simulink model "pmsm_mpc_ekf"  (R2025b)
settings: Solver=ode23tb  StartTime=0.0  StopTime=simlength  FixedStep=tsample  MaxStep=ts
undefined symbols (not defined in the file): A1_tilde, A2_tilde, A3_tilde, A4_tilde, Adrso, b, b_brake, Bd, C, Crso, ibez, Jm, ki_w, kp_w, Lalpha, Lbeta, Ldrso, omega_bez, omega_m_bez, omega_m_sim, psi_m, Qkalman, Rkalman, Rs, simlength, tau_bez, tcontrol, ts, Vdc
libraries: fl_lib x19, nesl_utility x19, pmsm_alphabeta_lib x1, psm x1
(part 1 of 2)
settings Model: SimulationMode=accelerator  Creator=dbagn  LastModifiedBy=dbagn
settings SolverCC: NumberNewtonIterations=3.0  ZeroCrossControl=DisableAll  AlgebraicLoopSolver=TrustRegion  SolverResetMethod=Robust
settings DataIOCC: ReturnWorkspaceOutputs=off
settings DebuggingCC: UnconnectedInputMsg=warning  UnconnectedOutputMsg=warning  UnconnectedLineMsg=warning
settings ModelReferenceCC: EnableRefExpFcnMdlSchedulingChecks=on
settings RTWCC: GPUComputeCapability=3.5  DLArmComputeVersion=19.05

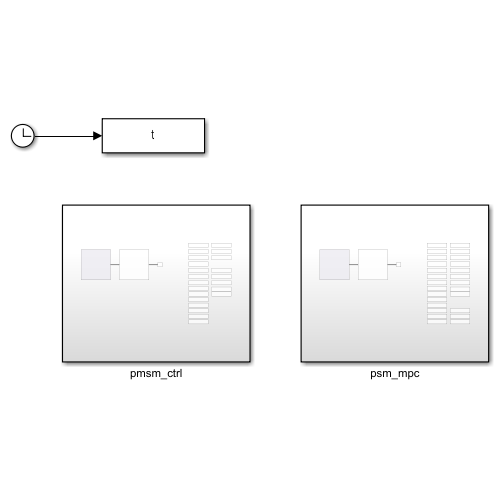
[thumbnail: Simulink's stored preview of the top-level diagram]
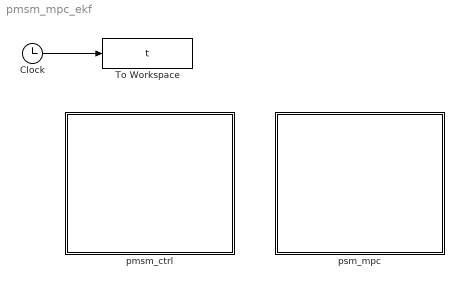
== system pmsm_mpc_ekf ==
  Clock : Clock
  To Workspace : ToWorkspace  VariableName=t  SampleTime=ts
      settings: MaxDataPoints=Nc
  pmsm_ctrl : Subsystem
  psm_mpc : Subsystem
  wires:
  Clock/1 -> To Workspace/1

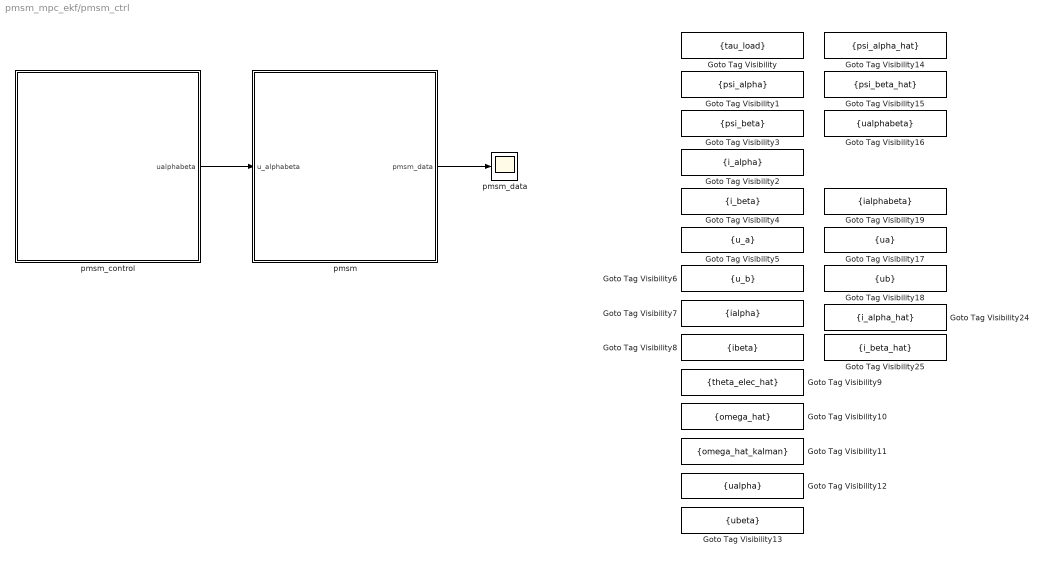
== system pmsm_mpc_ekf/pmsm_ctrl ==
  Goto Tag Visibility : GotoTagVisibility  GotoTag=tau_load
  Goto Tag Visibility1 : GotoTagVisibility  GotoTag=psi_alpha
  Goto Tag Visibility10 : GotoTagVisibility  GotoTag=omega_hat
  Goto Tag Visibility11 : GotoTagVisibility  GotoTag=omega_hat_kalman
  Goto Tag Visibility12 : GotoTagVisibility  GotoTag=ualpha
  Goto Tag Visibility13 : GotoTagVisibility  GotoTag=ubeta
  Goto Tag Visibility14 : GotoTagVisibility  GotoTag=psi_alpha_hat
  Goto Tag Visibility15 : GotoTagVisibility  GotoTag=psi_beta_hat
  Goto Tag Visibility16 : GotoTagVisibility  GotoTag=ualphabeta
  Goto Tag Visibility17 : GotoTagVisibility  GotoTag=ua
  Goto Tag Visibility18 : GotoTagVisibility  GotoTag=ub
  Goto Tag Visibility19 : GotoTagVisibility  GotoTag=ialphabeta
  Goto Tag Visibility2 : GotoTagVisibility  GotoTag=i_alpha
  Goto Tag Visibility24 : GotoTagVisibility  GotoTag=i_alpha_hat
  Goto Tag Visibility25 : GotoTagVisibility  GotoTag=i_beta_hat
  Goto Tag Visibility3 : GotoTagVisibility  GotoTag=psi_beta
  Goto Tag Visibility4 : GotoTagVisibility  GotoTag=i_beta
  Goto Tag Visibility5 : GotoTagVisibility  GotoTag=u_a
  Goto Tag Visibility6 : GotoTagVisibility  GotoTag=u_b
  Goto Tag Visibility7 : GotoTagVisibility  GotoTag=ialpha
  Goto Tag Visibility8 : GotoTagVisibility  GotoTag=ibeta
  Goto Tag Visibility9 : GotoTagVisibility  GotoTag=theta_elec_hat
  pmsm : Subsystem
  pmsm_control : Subsystem
  pmsm_data : Scope
      settings: ActiveDisplayYMinimum=-7553.3407677630657  ActiveDisplayYMaximum=8430.65022613591
  wires:
  pmsm_control/1(ualphabeta) -> pmsm/1(u_alphabeta)
  pmsm/1(pmsm_data) -> pmsm_data/1

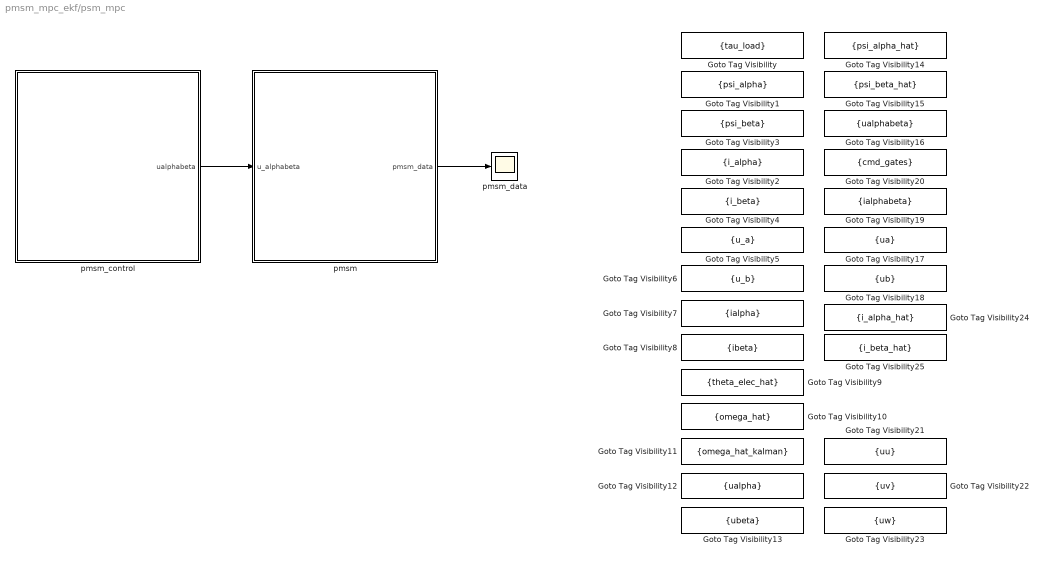
== system pmsm_mpc_ekf/psm_mpc ==
  Goto Tag Visibility : GotoTagVisibility  GotoTag=tau_load
  Goto Tag Visibility1 : GotoTagVisibility  GotoTag=psi_alpha
  Goto Tag Visibility10 : GotoTagVisibility  GotoTag=omega_hat
  Goto Tag Visibility11 : GotoTagVisibility  GotoTag=omega_hat_kalman
  Goto Tag Visibility12 : GotoTagVisibility  GotoTag=ualpha
  Goto Tag Visibility13 : GotoTagVisibility  GotoTag=ubeta
  Goto Tag Visibility14 : GotoTagVisibility  GotoTag=psi_alpha_hat
  Goto Tag Visibility15 : GotoTagVisibility  GotoTag=psi_beta_hat
  Goto Tag Visibility16 : GotoTagVisibility  GotoTag=ualphabeta
  Goto Tag Visibility17 : GotoTagVisibility  GotoTag=ua
  Goto Tag Visibility18 : GotoTagVisibility  GotoTag=ub
  Goto Tag Visibility19 : GotoTagVisibility  GotoTag=ialphabeta
  Goto Tag Visibility2 : GotoTagVisibility  GotoTag=i_alpha
  Goto Tag Visibility20 : GotoTagVisibility  GotoTag=cmd_gates
  Goto Tag Visibility21 : GotoTagVisibility  GotoTag=uu
  Goto Tag Visibility22 : GotoTagVisibility  GotoTag=uv
  Goto Tag Visibility23 : GotoTagVisibility  GotoTag=uw
  Goto Tag Visibility24 : GotoTagVisibility  GotoTag=i_alpha_hat
  Goto Tag Visibility25 : GotoTagVisibility  GotoTag=i_beta_hat
  Goto Tag Visibility3 : GotoTagVisibility  GotoTag=psi_beta
  Goto Tag Visibility4 : GotoTagVisibility  GotoTag=i_beta
  Goto Tag Visibility5 : GotoTagVisibility  GotoTag=u_a
  Goto Tag Visibility6 : GotoTagVisibility  GotoTag=u_b
  Goto Tag Visibility7 : GotoTagVisibility  GotoTag=ialpha
  Goto Tag Visibility8 : GotoTagVisibility  GotoTag=ibeta
  Goto Tag Visibility9 : GotoTagVisibility  GotoTag=theta_elec_hat
  pmsm : Subsystem
  pmsm_control : Subsystem
  pmsm_data : Scope
      settings: ActiveDisplayYMinimum=-7553.3407677630657  ActiveDisplayYMaximum=8430.65022613591
  wires:
  pmsm/1(pmsm_data) -> pmsm_data/1
  pmsm_control/1(ualphabeta) -> pmsm/1(u_alphabeta)

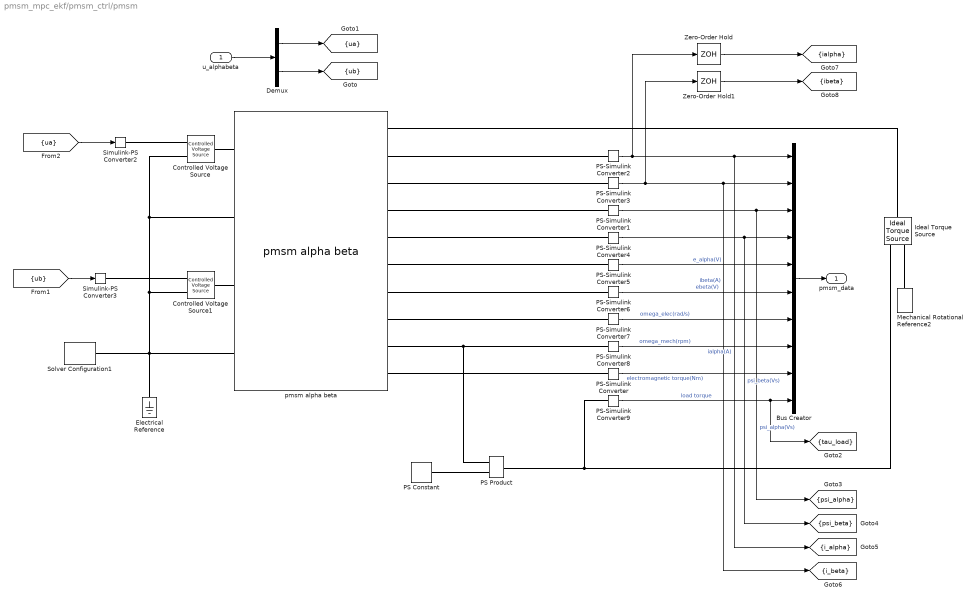
== system pmsm_mpc_ekf/pmsm_ctrl/pmsm ==
  u_alphabeta : Inport
  Bus Creator : BusCreator  Inputs=10
  Controlled Voltage Source : fl_lib/Electrical/Electrical Sources/Controlled Voltage Source
  Controlled Voltage Source1 : fl_lib/Electrical/Electrical Sources/Controlled Voltage Source
  Demux : Demux  Outputs=2
  Electrical Reference : fl_lib/Electrical/Electrical Elements/Electrical Reference
  Ideal Torque Source : fl_lib/Mechanical/Mechanical Sources/Ideal Torque Source
  Mechanical Rotational Reference2 : fl_lib/Mechanical/Rotational Elements/Mechanical Rotational Reference
  PS Constant : fl_lib/Physical Signals/Sources/PS Constant  constant=-b_brake N*m/(rad/s)
  PS Product : fl_lib/Physical Signals/Functions/PS Product
  PS-Simulink Converter : nesl_utility/PS-Simulink Converter  PhysicalDomain=network_engine_domain  SubClassName=ps_output  LeftPortType=input  RightPortType=output  PseudoPeriodic=off  Frequencies=[]  VectorFormat=1-D array  Unit=N*m  AffineConversion=on
  PS-Simulink Converter1 : nesl_utility/PS-Simulink Converter  PhysicalDomain=network_engine_domain  SubClassName=ps_output  LeftPortType=input  RightPortType=output  PseudoPeriodic=off  Frequencies=[]  VectorFormat=1-D array  Unit=V*s  AffineConversion=on
  PS-Simulink Converter2 : nesl_utility/PS-Simulink Converter  PhysicalDomain=network_engine_domain  SubClassName=ps_output  LeftPortType=input  RightPortType=output  PseudoPeriodic=off  Frequencies=[]  VectorFormat=1-D array  Unit=A  AffineConversion=on
  PS-Simulink Converter3 : nesl_utility/PS-Simulink Converter  PhysicalDomain=network_engine_domain  SubClassName=ps_output  LeftPortType=input  RightPortType=output  PseudoPeriodic=off  Frequencies=[]  VectorFormat=1-D array  Unit=A  AffineConversion=on
  PS-Simulink Converter4 : nesl_utility/PS-Simulink Converter  PhysicalDomain=network_engine_domain  SubClassName=ps_output  LeftPortType=input  RightPortType=output  PseudoPeriodic=off  Frequencies=[]  VectorFormat=1-D array  Unit=V*s  AffineConversion=on
  PS-Simulink Converter5 : nesl_utility/PS-Simulink Converter  PhysicalDomain=network_engine_domain  SubClassName=ps_output  LeftPortType=input  RightPortType=output  PseudoPeriodic=off  Frequencies=[]  VectorFormat=1-D array  Unit=V  AffineConversion=on
  PS-Simulink Converter6 : nesl_utility/PS-Simulink Converter  PhysicalDomain=network_engine_domain  SubClassName=ps_output  LeftPortType=input  RightPortType=output  PseudoPeriodic=off  Frequencies=[]  VectorFormat=1-D array  Unit=V  AffineConversion=on
  PS-Simulink Converter7 : nesl_utility/PS-Simulink Converter  PhysicalDomain=network_engine_domain  SubClassName=ps_output  LeftPortType=input  RightPortType=output  PseudoPeriodic=off  Frequencies=[]  VectorFormat=1-D array  Unit=rad/s  AffineConversion=on
  PS-Simulink Converter8 : nesl_utility/PS-Simulink Converter  PhysicalDomain=network_engine_domain  SubClassName=ps_output  LeftPortType=input  RightPortType=output  PseudoPeriodic=off  Frequencies=[]  VectorFormat=1-D array  Unit=rpm  AffineConversion=on
  PS-Simulink Converter9 : nesl_utility/PS-Simulink Converter  PhysicalDomain=network_engine_domain  SubClassName=ps_output  LeftPortType=input  RightPortType=output  PseudoPeriodic=off  Frequencies=[]  VectorFormat=1-D array  Unit=N*m  AffineConversion=on
  Simulink-PS Converter2 : nesl_utility/Simulink-PS Converter  PhysicalDomain=network_engine_domain  SubClassName=ps_input  LeftPortType=input  RightPortType=output  PseudoPeriodic=off  Frequencies=[]  NoiseDistribution=none  NoiseParameters=[]  Unit=1  AffineConversion=off  FilteringAndDerivatives=provide  SimscapeFilterOrder=1  InputFilterTimeConstant=0.001  UdotUserProvided=0
  Simulink-PS Converter3 : nesl_utility/Simulink-PS Converter  PhysicalDomain=network_engine_domain  SubClassName=ps_input  LeftPortType=input  RightPortType=output  PseudoPeriodic=off  Frequencies=[]  NoiseDistribution=none  NoiseParameters=[]  Unit=1  AffineConversion=off  FilteringAndDerivatives=provide  SimscapeFilterOrder=1  InputFilterTimeConstant=0.001  UdotUserProvided=0
  Solver Configuration1 : nesl_utility/Solver Configuration  PhysicalDomain=network_engine_domain  SubClassName=solver  LeftPortType=input  RightPortType=generic  Tones=[]  Harmonics=[]  SimulateNoise=off  Profile=off  UseLocalSampling=off  EnableSwitchedLinearOptims=on  FrequencyDomain=off  UseCCode=off  RelTol=0.001  AbsTol=1e-06  MinStep=1e-09  ToWorkspace=off  RevertToSquareIcSolve=off  NumHomotopyIterations=100  PhasorMode=off  PhasorModeNumHarmonics=1  ConsistencySolver=NEWTON_FTOL  IndexReductionMethod=DerivativeReplacement  DoDC=on  ResidualTolerance=1e-09  ConsistencyTolSource=GLOBAL  ConsistencyAbsTol=0.001  ConsistencyRelTol=0.001  ConsistencyTolFactor=0.001  UseLocalSolver=on  LocalSolverChoice=NE_TRAPEZOIDAL_ADVANCER  ResolveIndetEquations=on  FunctionEvalNumThread=1  LocalSolverSampleTime=ts  DoFixedCost=on  MaxNonlinIter=3  MaxModeIter=2  ComputeImpulses=off  ImpulseIterations=2  LinearAlgebra=auto  LinearAlgebraNumThread=0  EquationFormulation=NE_TIME_EF  DelaysMemoryBudget=1024*4  AutomaticFiltering=on  FilteringTimeConstant=ts  PartitionStorageMethod=AS_NEEDED  PartitionMemoryBudget=1024  PartitionMethod=ROBUST  MultibodyUseLocalSolver=off  MultibodyLocalSolverChoice=ODE1  MultibodyLocalSolverSampleTime=0.001
  Zero-Order Hold : ZeroOrderHold  SampleTime=tcontrol
  Zero-Order Hold1 : ZeroOrderHold  SampleTime=tcontrol
  pmsm alpha beta : pmsm_alphabeta_lib/pmsm alpha beta  number_poles=number_poles  psi_m=psi_m V*s  Ls=Ls H  Lb=Lb H  Rs=Rs Ohm  J=Jm kg*m^2  b=b N*m/(rad/s)  omega_specify=off  omega_priority=None  omega=0 rad/s  omega_nominal_specify=off  omega_nominal_unit=rad/s  omega_nominal_value=1  omega_m_specify=off  omega_m_priority=None  omega_m=0 rad/s  omega_m_nominal_specify=off  omega_m_nominal_unit=rad/s  omega_m_nominal_value=1  ialpha_specify=on  ialpha_priority=High  ialpha=0 A  ialpha_nominal_specify=off  ialpha_nominal_unit=A  ialpha_nominal_value=1  ualpha_specify=off  ualpha_priority=None  ualpha=0 V  ualpha_nominal_specify=off  ualpha_nominal_unit=V  ualpha_nominal_value=1  psi_beta_specify=off  psi_beta_priority=High  psi_beta=0.0 V*s  psi_beta_nominal_specify=off  psi_beta_nominal_unit=V*s  psi_beta_nominal_value=1  ibeta_specify=on  ibeta_priority=High  ibeta=0 A  ibeta_nominal_specify=off  ibeta_nominal_unit=A  ibeta_nominal_value=1  ubeta_specify=off  ubeta_priority=None  ubeta=0 V  ubeta_nominal_specify=off  ubeta_nominal_unit=V  ubeta_nominal_value=1  tau_load_specify=off  tau_load_priority=None  tau_load=0 N*m  tau_load_nominal_specify=off  tau_load_nominal_unit=N*m  tau_load_nominal_value=1
      settings: InternalSimscapePortConfiguration="{\"Bottom\":[],\"Left\":[{\"id\":\"u_alpha_p\",\"label\":\"_u_alpha+_\",\"type\":\"foundation.electrical.electrical\"},{\"id\":\"u_alpha_n\",\"label\":\"_u_alpha-_\",\"type\":\"foundation.electrical.electrical\"},{\"id\":\"u_beta_p\",\"label\":\"_u_beta+_\",\"type\":\"foundation.electrical.electrical\"},{\"id\":\"u_beta_n\",\"label\":\"_u_beta-_\",\"type\":\"foundation.electrical.electrical\"}],\"Right\":[{\"id\":\"s\",\"label\":\"_s_\",\"type\":\"foundation.mechanical.rotational.rotational\"},{\"id\":\"i_alpha_out\",\"label\":\"_i_alpha_\",\"type\":\"output\"},{\"id\":\"i_beta_out\",\"label\":\"_i_beta_\",\"type\":\"output\"},{\"id\":\"psi_alpha_out\",\"label\":\"_psi_alpha_\",\"type\":\"output\"},{\"id\":\"psi_beta_out\",\"label\":\"_psi_beta_\",\"type\":\"output\"},{\"id\":\"e_alpha_out\",\"label\":\"_e_alpha_\",\"type\":\"output\"},{\"id\":\"e_beta_out\",\"label\":\"_e_beta_\",\"type\":\"output\"},{\"id\":\"omega_elec_out\",\"label\":\"_omega_elec_\",\"type\":\"output\"},{\"id\":\"omega_mech_out\",\"label\":\"_omega_mech_\",\"type\":\"output\"},{\"id\":\"torque_e_out\",\"label\":\"_torque_e_\",\"type\":\"output\"}],\"Top\":[]}"
  pmsm_data : Outport
  tag scope: i_alpha=scoped, i_beta=scoped, ialpha=scoped, ibeta=scoped, psi_alpha=scoped, psi_beta=scoped, tau_load=scoped, ua=scoped, ub=scoped
  wires:
  [ua] -> Simulink-PS Converter2/1
  [ub] -> Simulink-PS Converter3/1
  u_alphabeta/1 -> Demux/1
  Demux/1 -> [ua]
  Demux/2 -> [ub]
  Zero-Order Hold/1 -> [ialpha]
  Zero-Order Hold1/1 -> [ibeta]
  PS-Simulink Converter2/1 -> [i_alpha], Bus Creator/1, Zero-Order Hold/1  "ialpha(A)"
  PS-Simulink Converter3/1 -> [i_beta], Bus Creator/2, Zero-Order Hold1/1  "ibeta(A)"
  PS-Simulink Converter1/1 -> [psi_alpha], Bus Creator/3  "psi_alpha(Vs)"
  PS-Simulink Converter4/1 -> Bus Creator/4, [psi_beta]  "psi_beta(Vs)"
  PS-Simulink Converter5/1 -> Bus Creator/5  "e_alpha(V)"
  PS-Simulink Converter6/1 -> Bus Creator/6  "ebeta(V)"
  PS-Simulink Converter7/1 -> Bus Creator/7  "omega_elec(rad/s)"
  PS-Simulink Converter8/1 -> Bus Creator/8  "omega_mech(rpm)"
  PS-Simulink Converter/1 -> Bus Creator/9  "electromagnetic torque(Nm)"
  PS-Simulink Converter9/1 -> Bus Creator/10, [tau_load]  "load torque"
  Bus Creator/1 -> pmsm_data/1
  connections:
  Controlled Voltage Source/RConn1 -- Simulink-PS Converter2/RConn1
  pmsm alpha beta/LConn1 -- Controlled Voltage Source/LConn1
  Simulink-PS Converter3/RConn1 -- Controlled Voltage Source1/RConn1
  pmsm alpha beta/LConn3 -- Controlled Voltage Source1/LConn1
  Controlled Voltage Source/RConn2 -- pmsm alpha beta/LConn2 -- Controlled Voltage Source1/RConn2 -- pmsm alpha beta/LConn4 -- Solver Configuration1/RConn1 -- Electrical Reference/LConn1
  pmsm alpha beta/RConn2 -- PS-Simulink Converter2/LConn1
  pmsm alpha beta/RConn3 -- PS-Simulink Converter3/LConn1
  PS-Simulink Converter4/LConn1 -- pmsm alpha beta/RConn5
  PS-Simulink Converter1/LConn1 -- pmsm alpha beta/RConn4
  PS-Simulink Converter5/LConn1 -- pmsm alpha beta/RConn6
  pmsm alpha beta/RConn7 -- PS-Simulink Converter6/LConn1
  Mechanical Rotational Reference2/LConn1 -- Ideal Torque Source/RConn2
  pmsm alpha beta/RConn1 -- Ideal Torque Source/LConn1
  pmsm alpha beta/RConn9 -- PS-Simulink Converter8/LConn1 -- PS Product/LConn1
  pmsm alpha beta/RConn10 -- PS-Simulink Converter/LConn1
  PS Constant/RConn1 -- PS Product/LConn2
  PS Product/RConn1 -- Ideal Torque Source/RConn1 -- PS-Simulink Converter9/LConn1
  pmsm alpha beta/RConn8 -- PS-Simulink Converter7/LConn1

== system pmsm_mpc_ekf/pmsm_ctrl/pmsm_control ==
  Mux : Mux  Inputs=2
  Speed control : Subsystem
  double_integrator_observer : Subsystem
  mpc_ekf : Subsystem
  normalization : Gain  Gain=1/omega_bez
  normalization1 : Gain  Gain=1/tau_bez
  omega_hat_kalman/omega_hat : Scope  NumInputPorts=2
      settings: SampleTime=tcontrol  ActiveDisplayYMinimum=-304.159  ActiveDisplayYMaximum=313.10699
  omega_ref/omega/torque load_pu : Scope  NumInputPorts=2
      settings: SampleTime=tcontrol  ActiveDisplayYMinimum=-1.08049  ActiveDisplayYMaximum=1.23758  DataLoggingVariableName=ScopeData3
  speed_reference_generator : Subsystem
  torque_ref_pu : Scope
      settings: SampleTime=tcontrol  ActiveDisplayYMinimum=-1.08049  ActiveDisplayYMaximum=1.23758
  ualphabeta : Outport  VectorParamsAs1DForOutWhenUnconnected=off
  tag scope: omega_hat=scoped
  wires:
  mpc_ekf/1(ualphabeta) -> ualphabeta/1
  normalization/1 -> Mux/1, Speed control/1(Rotor speed)  "omega_pu"
  [theta_elec_hat] -> double_integrator_observer/1(theta)
  Speed control/1(torque_ref_pu) -> torque_ref_pu/1, mpc_ekf/1(torque_ref_pu)  "torque_ref_pu"
  speed_reference_generator/1(omega_ref_pu) -> Speed control/2(Speed ref), Mux/2  "omega_ref_pu"
  Mux/1 -> omega_ref/omega/torque load_pu/1
  [tau_load] -> normalization1/1
  normalization1/1 -> omega_ref/omega/torque load_pu/2  "torque load_pu"
  double_integrator_observer/1(omega_hat) -> [omega_hat], normalization/1
  [omega_hat_kalman] -> omega_hat_kalman/omega_hat/1  "omega_hat_kalman"
  [omega_hat] -> omega_hat_kalman/omega_hat/2  "omega_hat"

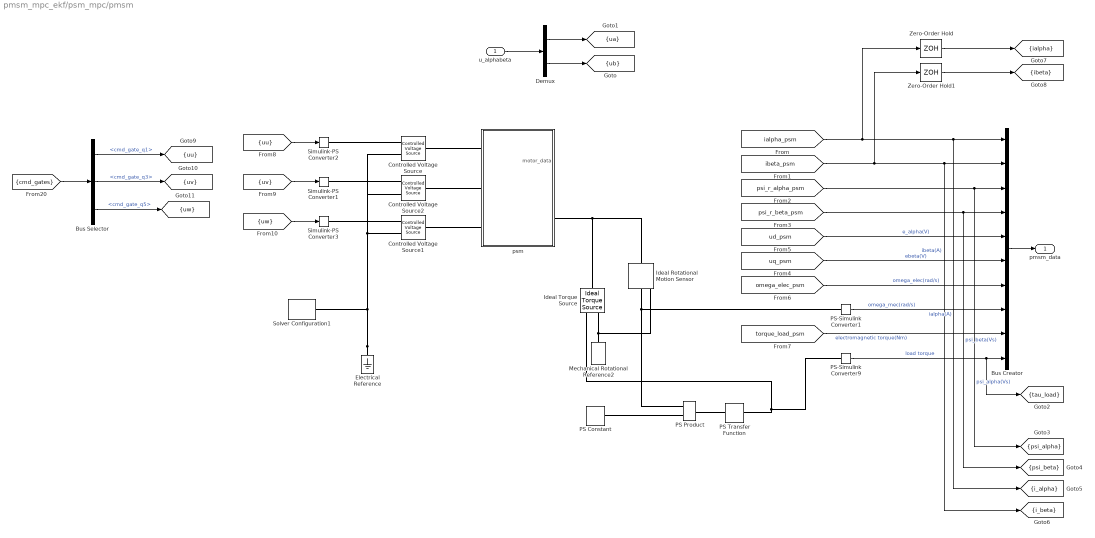
== system pmsm_mpc_ekf/psm_mpc/pmsm ==
  u_alphabeta : Inport
  Bus Creator : BusCreator  Inputs=10
  Bus Selector : BusSelector  OutputSignals=cmd_gate_q1,cmd_gate_q3,cmd_gate_q5
  Controlled Voltage Source : fl_lib/Electrical/Electrical Sources/Controlled Voltage Source
  Controlled Voltage Source1 : fl_lib/Electrical/Electrical Sources/Controlled Voltage Source
  Controlled Voltage Source2 : fl_lib/Electrical/Electrical Sources/Controlled Voltage Source
  Demux : Demux  Outputs=2
  Electrical Reference : fl_lib/Electrical/Electrical Elements/Electrical Reference
  Ideal Rotational Motion Sensor : fl_lib/Mechanical/Mechanical Sensors/Ideal Rotational Motion Sensor  reference=foundation.enum.MeasurementReference.difference  acceleration_port=false  velocity_port=true  position_port=true  wrap_angle=false  offset=0 rad
  Ideal Torque Source : fl_lib/Mechanical/Mechanical Sources/Ideal Torque Source
  Mechanical Rotational Reference2 : fl_lib/Mechanical/Rotational Elements/Mechanical Rotational Reference
  PS Constant : fl_lib/Physical Signals/Sources/PS Constant  constant=-b_brake N*m/(rad/s)
  PS Product : fl_lib/Physical Signals/Functions/PS Product
  PS Transfer Function : fl_lib/Physical Signals/Linear Operators/PS Transfer Function  transfer_function_type=foundation.enum.transfer_function_type.lag  T=0.05 s  T1=2 s  T2=1 s  reset_method=foundation.enum.IntegratorResetSpec.None  initial_condition_spec=foundation.enum.IntegratorICSpec.Internal  y0=0 N*m
      settings: InternalSimscapePortConfiguration="{\"Bottom\":[],\"Left\":[{\"id\":\"U\",\"label\":\"\",\"type\":\"input\"}],\"Right\":[{\"id\":\"Y\",\"label\":\"\",\"type\":\"output\"}],\"Top\":[]}"
  PS-Simulink Converter1 : nesl_utility/PS-Simulink Converter  PhysicalDomain=network_engine_domain  SubClassName=ps_output  LeftPortType=input  RightPortType=output  PseudoPeriodic=off  Frequencies=[]  VectorFormat=1-D array  Unit=rpm  AffineConversion=on
  PS-Simulink Converter9 : nesl_utility/PS-Simulink Converter  PhysicalDomain=network_engine_domain  SubClassName=ps_output  LeftPortType=input  RightPortType=output  PseudoPeriodic=off  Frequencies=[]  VectorFormat=1-D array  Unit=N*m  AffineConversion=on
  Simulink-PS Converter1 : nesl_utility/Simulink-PS Converter  PhysicalDomain=network_engine_domain  SubClassName=ps_input  LeftPortType=input  RightPortType=output  PseudoPeriodic=off  Frequencies=[]  NoiseDistribution=none  NoiseParameters=[]  Unit=1  AffineConversion=off  FilteringAndDerivatives=provide  SimscapeFilterOrder=1  InputFilterTimeConstant=0.001  UdotUserProvided=0
  Simulink-PS Converter2 : nesl_utility/Simulink-PS Converter  PhysicalDomain=network_engine_domain  SubClassName=ps_input  LeftPortType=input  RightPortType=output  PseudoPeriodic=off  Frequencies=[]  NoiseDistribution=none  NoiseParameters=[]  Unit=1  AffineConversion=off  FilteringAndDerivatives=provide  SimscapeFilterOrder=1  InputFilterTimeConstant=0.001  UdotUserProvided=0
  Simulink-PS Converter3 : nesl_utility/Simulink-PS Converter  PhysicalDomain=network_engine_domain  SubClassName=ps_input  LeftPortType=input  RightPortType=output  PseudoPeriodic=off  Frequencies=[]  NoiseDistribution=none  NoiseParameters=[]  Unit=1  AffineConversion=off  FilteringAndDerivatives=provide  SimscapeFilterOrder=1  InputFilterTimeConstant=0.001  UdotUserProvided=0
  Solver Configuration1 : nesl_utility/Solver Configuration  PhysicalDomain=network_engine_domain  SubClassName=solver  LeftPortType=input  RightPortType=generic  Tones=[]  Harmonics=[]  SimulateNoise=off  Profile=off  UseLocalSampling=off  EnableSwitchedLinearOptims=on  FrequencyDomain=off  UseCCode=off  RelTol=0.001  AbsTol=1e-06  MinStep=1e-09  ToWorkspace=off  RevertToSquareIcSolve=off  NumHomotopyIterations=100  PhasorMode=off  PhasorModeNumHarmonics=1  ConsistencySolver=NEWTON_FTOL  IndexReductionMethod=DerivativeReplacement  DoDC=on  ResidualTolerance=1e-09  ConsistencyTolSource=GLOBAL  ConsistencyAbsTol=0.001  ConsistencyRelTol=0.001  ConsistencyTolFactor=0.001  UseLocalSolver=on  LocalSolverChoice=NE_TRAPEZOIDAL_ADVANCER  ResolveIndetEquations=on  FunctionEvalNumThread=1  LocalSolverSampleTime=ts  DoFixedCost=on  MaxNonlinIter=3  MaxModeIter=2  ComputeImpulses=off  ImpulseIterations=2  LinearAlgebra=auto  LinearAlgebraNumThread=0  EquationFormulation=NE_TIME_EF  DelaysMemoryBudget=1024*4  AutomaticFiltering=on  FilteringTimeConstant=ts  PartitionStorageMethod=AS_NEEDED  PartitionMemoryBudget=1024  PartitionMethod=ROBUST  MultibodyUseLocalSolver=off  MultibodyLocalSolverChoice=ODE1  MultibodyLocalSolverSampleTime=0.001
  Zero-Order Hold : ZeroOrderHold  SampleTime=tcontrol
  Zero-Order Hold1 : ZeroOrderHold  SampleTime=tcontrol
  psm : Subsystem
  pmsm_data : Outport
  tag scope: i_alpha=scoped, i_beta=scoped, ialpha=scoped, ibeta=scoped, psi_alpha=scoped, psi_beta=scoped, tau_load=scoped, ua=scoped, ub=scoped, uu=scoped, uv=scoped, uw=scoped
  wires:
  Bus Creator/1 -> pmsm_data/1
  PS-Simulink Converter9/1 -> [tau_load], Bus Creator/10  "load torque"
  [torque_load_psm] -> Bus Creator/9  "electromagnetic torque(Nm)"
  [omega_elec_psm] -> Bus Creator/7  "omega_elec(rad/s)"
  [uq_psm] -> Bus Creator/6  "ebeta(V)"
  [ud_psm] -> Bus Creator/5  "e_alpha(V)"
  [psi_r_beta_psm] -> [psi_beta], Bus Creator/4  "psi_beta(Vs)"
  [psi_r_alpha_psm] -> Bus Creator/3, [psi_alpha]  "psi_alpha(Vs)"
  [ibeta_psm] -> Zero-Order Hold1/1, Bus Creator/2, [i_beta]  "ibeta(A)"
  [ialpha_psm] -> Zero-Order Hold/1, Bus Creator/1, [i_alpha]  "ialpha(A)"
  Zero-Order Hold1/1 -> [ibeta]
  Zero-Order Hold/1 -> [ialpha]
  Demux/2 -> [ub]
  Demux/1 -> [ua]
  u_alphabeta/1 -> Demux/1
  [cmd_gates] -> Bus Selector/1
  Bus Selector/1 -> [uu]  "<cmd_gate_q1>"
  Bus Selector/3 -> [uw]  "<cmd_gate_q5>"
  Bus Selector/2 -> [uv]  "<cmd_gate_q3>"
  [uu] -> Simulink-PS Converter2/1
  [uv] -> Simulink-PS Converter1/1
  [uw] -> Simulink-PS Converter3/1
  PS-Simulink Converter1/1 -> Bus Creator/8  "omega_mec(rad/s)"
  connections:
  PS Product/RConn1 -- PS Transfer Function/LConn1
  PS Constant/RConn1 -- PS Product/LConn2
  Mechanical Rotational Reference2/LConn1 -- Ideal Rotational Motion Sensor/RConn1 -- Ideal Torque Source/RConn2
  Electrical Reference/LConn1 -- Solver Configuration1/RConn1 -- Controlled Voltage Source/RConn2 -- Controlled Voltage Source2/RConn2 -- Controlled Voltage Source1/RConn2
  Controlled Voltage Source1/LConn1 -- psm/LConn3
  Simulink-PS Converter3/RConn1 -- Controlled Voltage Source1/RConn1
  Controlled Voltage Source/LConn1 -- psm/LConn1
  Controlled Voltage Source/RConn1 -- Simulink-PS Converter2/RConn1
  Simulink-PS Converter1/RConn1 -- Controlled Voltage Source2/RConn1
  psm/LConn2 -- Controlled Voltage Source2/LConn1
  Ideal Torque Source/LConn1 -- psm/RConn1 -- Ideal Rotational Motion Sensor/LConn1
  Ideal Rotational Motion Sensor/RConn2 -- PS Product/LConn1 -- PS-Simulink Converter1/LConn1
  PS Transfer Function/RConn1 -- PS-Simulink Converter9/LConn1 -- Ideal Torque Source/RConn1

== system pmsm_mpc_ekf/psm_mpc/pmsm_control ==
  Mux : Mux  Inputs=2
  Speed control : Subsystem
  double_integrator_observer : Subsystem
  mpc_ekf : Subsystem
  normalization : Gain  Gain=1/omega_bez
  normalization1 : Gain  Gain=1/tau_bez
  omega_hat_kalman/omega_hat : Scope  NumInputPorts=2
      settings: SampleTime=tcontrol  ActiveDisplayYMinimum=-304.159  ActiveDisplayYMaximum=313.10699
  omega_ref/omega/torque load_pu : Scope  NumInputPorts=2
      settings: SampleTime=tcontrol  ActiveDisplayYMinimum=-1.08049  ActiveDisplayYMaximum=1.23758  DataLoggingVariableName=ScopeData3
  speed_reference_generator : Subsystem
  torque_ref_pu : Scope
      settings: SampleTime=tcontrol  ActiveDisplayYMinimum=-1.08049  ActiveDisplayYMaximum=1.23758
  ualphabeta : Outport  VectorParamsAs1DForOutWhenUnconnected=off
  tag scope: omega_hat=scoped
  wires:
  [omega_hat] -> omega_hat_kalman/omega_hat/2  "omega_hat"
  [omega_hat_kalman] -> omega_hat_kalman/omega_hat/1  "omega_hat_kalman"
  double_integrator_observer/1(omega_hat) -> normalization/1, [omega_hat]
  normalization1/1 -> omega_ref/omega/torque load_pu/2  "torque load_pu"
  [tau_load] -> normalization1/1
  Mux/1 -> omega_ref/omega/torque load_pu/1
  speed_reference_generator/1(omega_ref_pu) -> Mux/2, Speed control/2(Speed ref)  "omega_ref_pu"
  Speed control/1(torque_ref_pu) -> mpc_ekf/1(torque_ref_pu), torque_ref_pu/1  "torque_ref_pu"
  [theta_elec_hat] -> double_integrator_observer/1(theta)
  normalization/1 -> Speed control/1(Rotor speed), Mux/1  "omega_pu"
  mpc_ekf/1(ualphabeta) -> ualphabeta/1

== system pmsm_mpc_ekf/pmsm_ctrl/pmsm_control/Speed control ==
  Rotor speed : Inport
  Speed ref : Inport  Port=2
  1/Ti : Gain  Gain=kp_w  SaturateOnIntegerOverflow=on  OutDataTypeStr=Inherit: Same as input  ParamDataTypeStr=Inherit: Same as input
  Saturation : Saturate  UpperLimit=1.5  LowerLimit=-1.5
  Sum1 : Sum  Inputs=+++  SaturateOnIntegerOverflow=on
  Sum2 : Sum  Inputs=-+  SaturateOnIntegerOverflow=on
  Sum3 : Sum  Inputs=-+  SaturateOnIntegerOverflow=on
  Unit Delay4 : UnitDelay  SampleTime=tcontrol  HasFrameUpgradeWarning=on
  kp : Gain  Gain=ki_w*tcontrol  SaturateOnIntegerOverflow=on  OutDataTypeStr=Inherit: Same as input  ParamDataTypeStr=Inherit: Same as input
  torque_ref_pu : Outport
  wires:
  1/Ti/1 -> Sum1/1, Sum3/1
  kp/1 -> Sum1/2
  Sum3/1 -> Unit Delay4/1
  Unit Delay4/1 -> Sum1/3
  Speed ref/1 -> Sum2/2
  Rotor speed/1 -> Sum2/1
  Sum2/1 -> kp/1, 1/Ti/1
  Saturation/1 -> torque_ref_pu/1, Sum3/2
  Sum1/1 -> Saturation/1

== system pmsm_mpc_ekf/pmsm_ctrl/pmsm_control/double_integrator_observer ==
  theta : Inport
  Gain : Gain  Gain=Ldrso  Multiplication=Matrix(K*u)
  Gain1 : Gain  Gain=Adrso  Multiplication=Matrix(K*u)
  Gain2 : Gain  Gain=Crso  Multiplication=Matrix(K*u)
  Selector : Selector  InputPortWidth=2  IndexOptions=Index vector (dialog)  Indices=2  OutputSizes=1
  Sum : Sum  Inputs=-+|
  Sum1 : Sum  Inputs=|++
  Unit Delay : UnitDelay  SampleTime=tcontrol  HasFrameUpgradeWarning=on
  Zero-Order Hold : ZeroOrderHold  SampleTime=tcontrol
  bounder1 : MATLAB Function  TreatAsAtomicUnit=on  SystemSampleTime=tcontrol
  bounder2 : MATLAB Function  TreatAsAtomicUnit=on  SystemSampleTime=tcontrol
  theta/theta_hat : Scope  NumInputPorts=2
      settings: SampleTime=ts  ActiveDisplayYMinimum=-3.92697  ActiveDisplayYMaximum=3.92696  DataLoggingVariableName=ScopeData3
  omega_hat : Outport
  wires:
  Gain/1 -> Sum1/1
  Selector/1 -> omega_hat/1
  Gain2/1 -> bounder2/1(u)  "theta_hat"
  Gain1/1 -> Sum1/2
  Sum1/1 -> Unit Delay/1
  Sum/1 -> bounder1/1(u)  "e"
  Unit Delay/1 -> Gain1/1, Selector/1, Gain2/1
  theta/1 -> Zero-Order Hold/1  "theta"
  Zero-Order Hold/1 -> theta/theta_hat/1, Sum/2  "theta_dsp"
  bounder1/1(y) -> Gain/1  "e_bounded"
  bounder2/1(y) -> theta/theta_hat/2, Sum/1  "theta_hat_bounded"

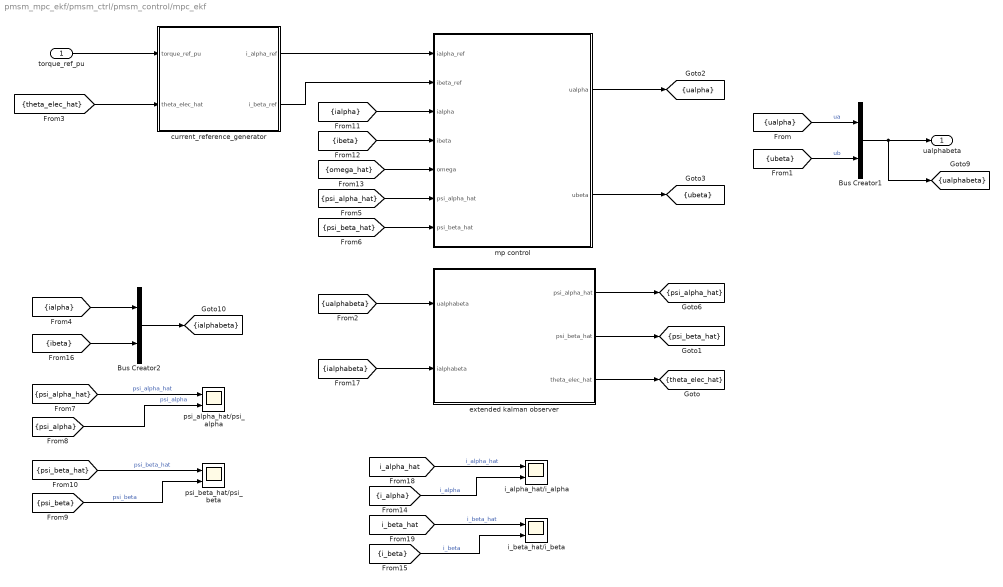
== system pmsm_mpc_ekf/pmsm_ctrl/pmsm_control/mpc_ekf ==
  torque_ref_pu : Inport
  Bus Creator1 : BusCreator  Inputs=2
  Bus Creator2 : BusCreator  Inputs=2
  current_reference_generator : Subsystem
  extended kalman observer : Subsystem
  i_alpha_hat/i_alpha : Scope  NumInputPorts=2
      settings: SampleTime=ts  ActiveDisplayYMinimum=-1380.23399  ActiveDisplayYMaximum=1473.77669  DataLoggingVariableName=ScopeData4
  i_beta_hat/i_beta : Scope  NumInputPorts=2
      settings: SampleTime=ts  ActiveDisplayYMinimum=610.865414775854  ActiveDisplayYMaximum=1049.3108922598913  DataLoggingVariableName=ScopeData5
  mp control : Subsystem
  psi_alpha_hat/psi_alpha : Scope  NumInputPorts=2
      settings: SampleTime=ts  ActiveDisplayYMinimum=-2.7502494573144358  ActiveDisplayYMaximum=2.7502552038903394  DataLoggingVariableName=ScopeData2
  psi_beta_hat/psi_beta : Scope  NumInputPorts=2
      settings: SampleTime=ts  ActiveDisplayYMinimum=-2.51196  ActiveDisplayYMaximum=2.51194  DataLoggingVariableName=ScopeData3
  ualphabeta : Outport  VectorParamsAs1DForOutWhenUnconnected=off
  tag scope: ialphabeta=scoped, psi_alpha_hat=scoped, psi_beta_hat=scoped, theta_elec_hat=scoped, ualpha=scoped, ualphabeta=scoped, ubeta=scoped
  wires:
  [ubeta] -> Bus Creator1/2  "ub"
  [ualpha] -> Bus Creator1/1  "ua"
  Bus Creator1/1 -> [ualphabeta], ualphabeta/1
  torque_ref_pu/1 -> current_reference_generator/1(torque_ref_pu)
  mp control/2(ubeta) -> [ubeta]
  mp control/1(ualpha) -> [ualpha]
  extended kalman observer/1(psi_alpha_hat) -> [psi_alpha_hat]
  extended kalman observer/2(psi_beta_hat) -> [psi_beta_hat]
  [psi_alpha_hat] -> mp control/6(psi_alpha_hat)
  [psi_beta_hat] -> mp control/7(psi_beta_hat)
  [ialpha] -> mp control/3(ialpha)
  [ibeta] -> mp control/4(ibeta)
  [omega_hat] -> mp control/5(omega)
  current_reference_generator/1(i_alpha_ref) -> mp control/1(ialpha_ref)
  current_reference_generator/2(i_beta_ref) -> mp control/2(ibeta_ref)
  [ualphabeta] -> extended kalman observer/1(ualphabeta)
  [ialpha] -> Bus Creator2/1
  [ibeta] -> Bus Creator2/2
  Bus Creator2/1 -> [ialphabeta]
  [ialphabeta] -> extended kalman observer/2(ialphabeta)
  [theta_elec_hat] -> current_reference_generator/2(theta_elec_hat)
  extended kalman observer/3(theta_elec_hat) -> [theta_elec_hat]
  [psi_alpha_hat] -> psi_alpha_hat/psi_alpha/1  "psi_alpha_hat"
  [psi_alpha] -> psi_alpha_hat/psi_alpha/2  "psi_alpha"
  [psi_beta_hat] -> psi_beta_hat/psi_beta/1  "psi_beta_hat"
  [psi_beta] -> psi_beta_hat/psi_beta/2  "psi_beta"
  [i_alpha_hat] -> i_alpha_hat/i_alpha/1  "i_alpha_hat"
  [i_alpha] -> i_alpha_hat/i_alpha/2  "i_alpha"
  [i_beta_hat] -> i_beta_hat/i_beta/1  "i_beta_hat"
  [i_beta] -> i_beta_hat/i_beta/2  "i_beta"

== system pmsm_mpc_ekf/pmsm_ctrl/pmsm_control/speed_reference_generator ==
  Rate Limiter : RateLimiter  RisingSlewLimit=0.25  FallingSlewLimit=-0.25  SampleTimeMode=inherited
  Step : Step  Time=simlength/20  After=omega_m_sim/omega_m_bez  SampleTime=0
  Step1 : Step  Time=simlength/2  After=-2*omega_m_sim/omega_m_bez  SampleTime=0
  Sum : Sum  Inputs=|++
  Transfer Fcn6 : TransferFcn  Numerator=[4]  Denominator=[1 4 4]
  omega_ref_pu : Outport
  wires:
  Rate Limiter/1 -> Transfer Fcn6/1
  Step/1 -> Sum/1
  Transfer Fcn6/1 -> omega_ref_pu/1
  Sum/1 -> Rate Limiter/1
  Step1/1 -> Sum/2

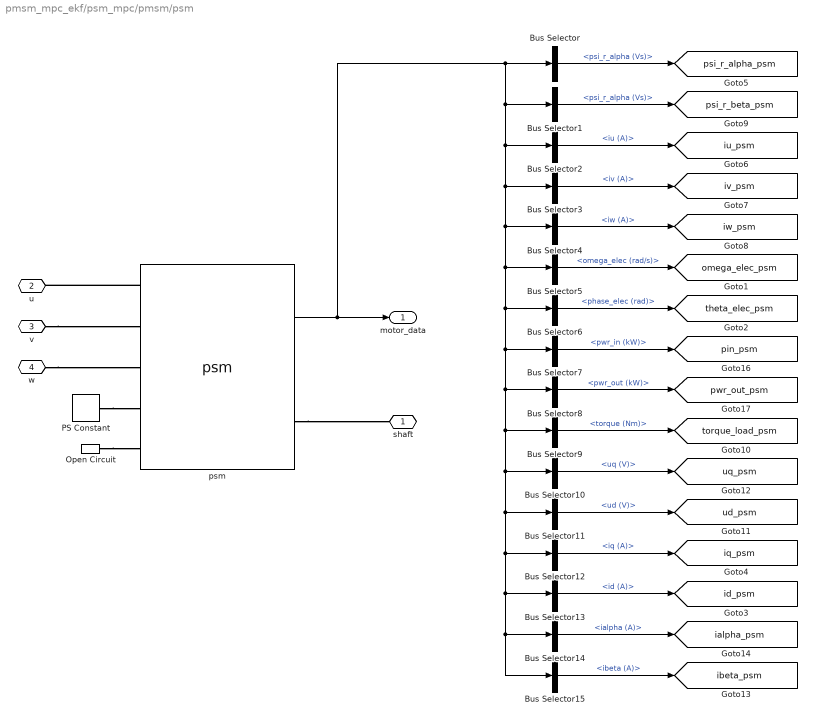
== system pmsm_mpc_ekf/psm_mpc/pmsm/psm ==
  Bus Selector : BusSelector  OutputSignals=psi_r_alpha (Vs)
  Bus Selector1 : BusSelector  OutputSignals=psi_r_alpha (Vs)
  Bus Selector10 : BusSelector  OutputSignals=uq (V)
  Bus Selector11 : BusSelector  OutputSignals=ud (V)
  Bus Selector12 : BusSelector  OutputSignals=iq (A)
  Bus Selector13 : BusSelector  OutputSignals=id (A)
  Bus Selector14 : BusSelector  OutputSignals=ialpha (A)
  Bus Selector15 : BusSelector  OutputSignals=ibeta (A)
  Bus Selector2 : BusSelector  OutputSignals=iu (A)
  Bus Selector3 : BusSelector  OutputSignals=iv (A)
  Bus Selector4 : BusSelector  OutputSignals=iw (A)
  Bus Selector5 : BusSelector  OutputSignals=omega_elec (rad/s)
  Bus Selector6 : BusSelector  OutputSignals=phase_elec (rad)
  Bus Selector7 : BusSelector  OutputSignals=pwr_in (kW)
  Bus Selector8 : BusSelector  OutputSignals=pwr_out (kW)
  Bus Selector9 : BusSelector  OutputSignals=torque (Nm)
  Open Circuit : fl_lib/Electrical/Electrical Elements/Open Circuit  v_specify=off  v_priority=None  v=0 V  v_nominal_specify=off  v_nominal_value=1  v_nominal_unit=V
  PS Constant : fl_lib/Physical Signals/Sources/PS Constant  constant=psi_m V*s
  psm : psm/psm  pp=number_poles  psi_m=psi_m  Lmu=5e-6  La=La  Lb=Lb  Rs=Rs  Jm=Jm  b_linear=b  b_quadratic=0  h5_percent=0  h7_percent=0  psi_r_u_init=psi_m  psi_r_v_init=-psi_m/2  psi_r_w_init=-psi_m/2
  shaft : PMIOPort  Side=Right
  u : PMIOPort  Port=2  Side=Left
  v : PMIOPort  Port=3  Side=Left
  w : PMIOPort  Port=4  Side=Left
  motor_data : Outport
  tag scope: ialpha_psm=global, ibeta_psm=global, id_psm=global, iq_psm=global, iu_psm=global, iv_psm=global, iw_psm=global, omega_elec_psm=global, pin_psm=global, psi_r_alpha_psm=global, psi_r_beta_psm=global, pwr_out_psm=global, theta_elec_psm=global, torque_load_psm=global, ud_psm=global, uq_psm=global
  wires:
  Bus Selector3/1 -> [iv_psm]  "<iv (A)>"
  Bus Selector6/1 -> [theta_elec_psm]  "<phase_elec (rad)>"
  Bus Selector5/1 -> [omega_elec_psm]  "<omega_elec (rad/s)>"
  Bus Selector12/1 -> [iq_psm]  "<iq (A)>"
  Bus Selector13/1 -> [id_psm]  "<id (A)>"
  Bus Selector1/1 -> [psi_r_beta_psm]  "<psi_r_alpha (Vs)>"
  Bus Selector10/1 -> [uq_psm]  "<uq (V)>"
  Bus Selector7/1 -> [pin_psm]  "<pwr_in (kW)>"
  Bus Selector8/1 -> [pwr_out_psm]  "<pwr_out (kW)>"
  Bus Selector4/1 -> [iw_psm]  "<iw (A)>"
  Bus Selector9/1 -> [torque_load_psm]  "<torque (Nm)>"
  Bus Selector/1 -> [psi_r_alpha_psm]  "<psi_r_alpha (Vs)>"
  Bus Selector11/1 -> [ud_psm]  "<ud (V)>"
  Bus Selector2/1 -> [iu_psm]  "<iu (A)>"
  Bus Selector15/1 -> [ibeta_psm]  "<ibeta (A)>"
  Bus Selector14/1 -> [ialpha_psm]  "<ialpha (A)>"
  psm/1 -> motor_data/1, Bus Selector8/1, Bus Selector10/1, Bus Selector11/1, Bus Selector12/1, Bus Selector14/1, Bus Selector15/1, Bus Selector13/1, Bus Selector9/1, Bus Selector7/1, Bus Selector6/1, Bus Selector5/1, Bus Selector4/1, Bus Selector3/1, Bus Selector2/1, Bus Selector1/1, Bus Selector/1
  connections:
  psm/RConn1 -- shaft/RConn1
  Open Circuit/LConn1 -- psm/LConn5
  v/RConn1 -- psm/LConn2
  psm/LConn1 -- u/RConn1
  w/RConn1 -- psm/LConn3
  PS Constant/RConn1 -- psm/LConn4

== system pmsm_mpc_ekf/psm_mpc/pmsm_control/Speed control ==
  Rotor speed : Inport
  Speed ref : Inport  Port=2
  1/Ti : Gain  Gain=kp_w  SaturateOnIntegerOverflow=on  OutDataTypeStr=Inherit: Same as input  ParamDataTypeStr=Inherit: Same as input
  Saturation : Saturate  UpperLimit=1.5  LowerLimit=-1.5
  Sum1 : Sum  Inputs=+++  SaturateOnIntegerOverflow=on
  Sum2 : Sum  Inputs=-+  SaturateOnIntegerOverflow=on
  Sum3 : Sum  Inputs=-+  SaturateOnIntegerOverflow=on
  Unit Delay4 : UnitDelay  SampleTime=tcontrol  HasFrameUpgradeWarning=on
  kp : Gain  Gain=ki_w*tcontrol  SaturateOnIntegerOverflow=on  OutDataTypeStr=Inherit: Same as input  ParamDataTypeStr=Inherit: Same as input
  torque_ref_pu : Outport
  wires:
  Sum1/1 -> Saturation/1
  Saturation/1 -> Sum3/2, torque_ref_pu/1
  Sum2/1 -> 1/Ti/1, kp/1
  Rotor speed/1 -> Sum2/1
  Speed ref/1 -> Sum2/2
  Unit Delay4/1 -> Sum1/3
  Sum3/1 -> Unit Delay4/1
  kp/1 -> Sum1/2
  1/Ti/1 -> Sum3/1, Sum1/1

== system pmsm_mpc_ekf/psm_mpc/pmsm_control/double_integrator_observer ==
  theta : Inport
  Gain : Gain  Gain=Ldrso  Multiplication=Matrix(K*u)
  Gain1 : Gain  Gain=Adrso  Multiplication=Matrix(K*u)
  Gain2 : Gain  Gain=Crso  Multiplication=Matrix(K*u)
  Selector : Selector  InputPortWidth=2  IndexOptions=Index vector (dialog)  Indices=2  OutputSizes=1
  Sum : Sum  Inputs=-+|
  Sum1 : Sum  Inputs=|++
  Unit Delay : UnitDelay  SampleTime=tcontrol  HasFrameUpgradeWarning=on
  Zero-Order Hold : ZeroOrderHold  SampleTime=tcontrol
  bounder1 : MATLAB Function  TreatAsAtomicUnit=on  SystemSampleTime=tcontrol
  bounder2 : MATLAB Function  TreatAsAtomicUnit=on  SystemSampleTime=tcontrol
  theta/theta_hat : Scope  NumInputPorts=2
      settings: SampleTime=ts  ActiveDisplayYMinimum=-3.92697  ActiveDisplayYMaximum=3.92696  DataLoggingVariableName=ScopeData3
  omega_hat : Outport
  wires:
  bounder2/1(y) -> Sum/1, theta/theta_hat/2  "theta_hat_bounded"
  bounder1/1(y) -> Gain/1  "e_bounded"
  Zero-Order Hold/1 -> Sum/2, theta/theta_hat/1  "theta_dsp"
  theta/1 -> Zero-Order Hold/1  "theta"
  Unit Delay/1 -> Gain2/1, Selector/1, Gain1/1
  Sum/1 -> bounder1/1(u)  "e"
  Sum1/1 -> Unit Delay/1
  Gain1/1 -> Sum1/2
  Gain2/1 -> bounder2/1(u)  "theta_hat"
  Selector/1 -> omega_hat/1
  Gain/1 -> Sum1/1

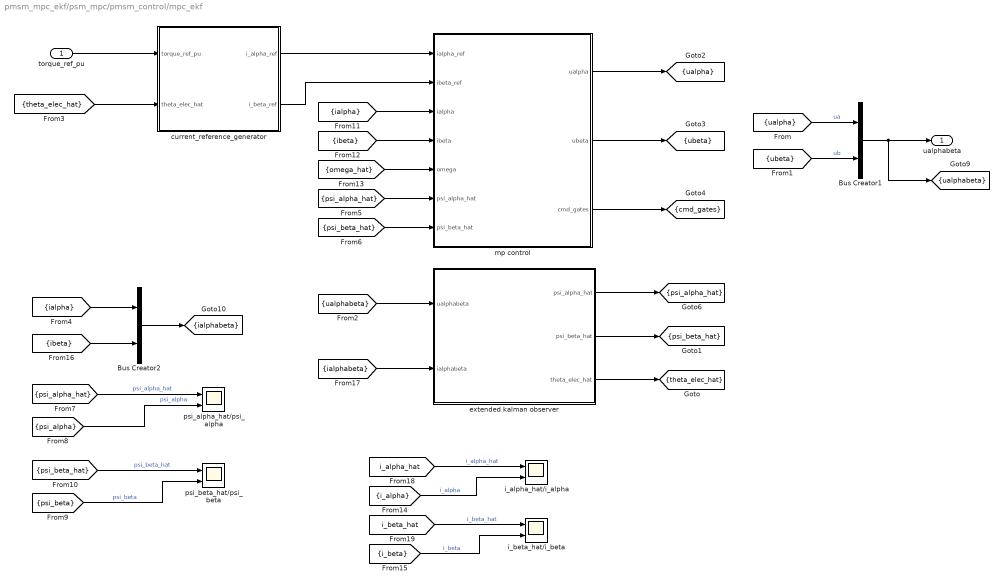
== system pmsm_mpc_ekf/psm_mpc/pmsm_control/mpc_ekf ==
  torque_ref_pu : Inport
  Bus Creator1 : BusCreator  Inputs=2
  Bus Creator2 : BusCreator  Inputs=2
  current_reference_generator : Subsystem
  extended kalman observer : Subsystem
  i_alpha_hat/i_alpha : Scope  NumInputPorts=2
      settings: SampleTime=ts  ActiveDisplayYMinimum=-1380.23399  ActiveDisplayYMaximum=1473.77669  DataLoggingVariableName=ScopeData4
  i_beta_hat/i_beta : Scope  NumInputPorts=2
      settings: SampleTime=ts  ActiveDisplayYMinimum=610.865414775854  ActiveDisplayYMaximum=1049.3108922598913  DataLoggingVariableName=ScopeData5
  mp control : Subsystem
  psi_alpha_hat/psi_alpha : Scope  NumInputPorts=2
      settings: SampleTime=ts  ActiveDisplayYMinimum=-2.7502494573144358  ActiveDisplayYMaximum=2.7502552038903394  DataLoggingVariableName=ScopeData2
  psi_beta_hat/psi_beta : Scope  NumInputPorts=2
      settings: SampleTime=ts  ActiveDisplayYMinimum=-2.51196  ActiveDisplayYMaximum=2.51194  DataLoggingVariableName=ScopeData3
  ualphabeta : Outport  VectorParamsAs1DForOutWhenUnconnected=off
  tag scope: cmd_gates=scoped, ialphabeta=scoped, psi_alpha_hat=scoped, psi_beta_hat=scoped, theta_elec_hat=scoped, ualpha=scoped, ualphabeta=scoped, ubeta=scoped
  wires:
  [i_beta] -> i_beta_hat/i_beta/2  "i_beta"
  [i_beta_hat] -> i_beta_hat/i_beta/1  "i_beta_hat"
  [i_alpha] -> i_alpha_hat/i_alpha/2  "i_alpha"
  [i_alpha_hat] -> i_alpha_hat/i_alpha/1  "i_alpha_hat"
  [psi_beta] -> psi_beta_hat/psi_beta/2  "psi_beta"
  [psi_beta_hat] -> psi_beta_hat/psi_beta/1  "psi_beta_hat"
  [psi_alpha] -> psi_alpha_hat/psi_alpha/2  "psi_alpha"
  [psi_alpha_hat] -> psi_alpha_hat/psi_alpha/1  "psi_alpha_hat"
  extended kalman observer/3(theta_elec_hat) -> [theta_elec_hat]
  [theta_elec_hat] -> current_reference_generator/2(theta_elec_hat)
  [ialphabeta] -> extended kalman observer/2(ialphabeta)
  Bus Creator2/1 -> [ialphabeta]
  [ibeta] -> Bus Creator2/2
  [ialpha] -> Bus Creator2/1
  [ualphabeta] -> extended kalman observer/1(ualphabeta)
  current_reference_generator/2(i_beta_ref) -> mp control/2(ibeta_ref)
  current_reference_generator/1(i_alpha_ref) -> mp control/1(ialpha_ref)
  [omega_hat] -> mp control/5(omega)
  [ibeta] -> mp control/4(ibeta)
  [ialpha] -> mp control/3(ialpha)
  [psi_beta_hat] -> mp control/7(psi_beta_hat)
  [psi_alpha_hat] -> mp control/6(psi_alpha_hat)
  extended kalman observer/2(psi_beta_hat) -> [psi_beta_hat]
  extended kalman observer/1(psi_alpha_hat) -> [psi_alpha_hat]
  mp control/1(ualpha) -> [ualpha]
  mp control/2(ubeta) -> [ubeta]
  torque_ref_pu/1 -> current_reference_generator/1(torque_ref_pu)
  Bus Creator1/1 -> ualphabeta/1, [ualphabeta]
  [ualpha] -> Bus Creator1/1  "ua"
  [ubeta] -> Bus Creator1/2  "ub"
  mp control/3(cmd_gates) -> [cmd_gates]

== system pmsm_mpc_ekf/psm_mpc/pmsm_control/speed_reference_generator ==
  Rate Limiter : RateLimiter  RisingSlewLimit=0.25  FallingSlewLimit=-0.25  SampleTimeMode=inherited
  Step : Step  Time=simlength/20  After=omega_m_sim/omega_m_bez  SampleTime=0
  Step1 : Step  Time=simlength/2  After=-2*omega_m_sim/omega_m_bez  SampleTime=0
  Sum : Sum  Inputs=|++
  Transfer Fcn6 : TransferFcn  Numerator=[4]  Denominator=[1 4 4]
  omega_ref_pu : Outport
  wires:
  Step1/1 -> Sum/2
  Sum/1 -> Rate Limiter/1
  Transfer Fcn6/1 -> omega_ref_pu/1
  Step/1 -> Sum/1
  Rate Limiter/1 -> Transfer Fcn6/1

== system pmsm_mpc_ekf/pmsm_ctrl/pmsm_control/mpc_ekf/current_reference_generator ==
  torque_ref_pu : Inport
  theta_elec_hat : Inport  Port=2
  Gain5 : Gain  Gain=-1
  Gain6 : Gain  Gain=ibez
  Product : Product
  Product1 : Product
  Trigonometric Function1 : Trigonometry
  Trigonometric Function2 : Trigonometry  Operator=cos
  i_alpha_ref : Outport
  i_beta_ref : Outport  Port=2
  wires:
  theta_elec_hat/1 -> Trigonometric Function2/1, Trigonometric Function1/1  "theta_electrical"
  Gain6/1 -> Product1/1, Product/1
  Gain5/1 -> i_alpha_ref/1
  Product/1 -> Gain5/1
  Trigonometric Function2/1 -> Product1/2
  Product1/1 -> i_beta_ref/1
  Trigonometric Function1/1 -> Product/2
  torque_ref_pu/1 -> Gain6/1

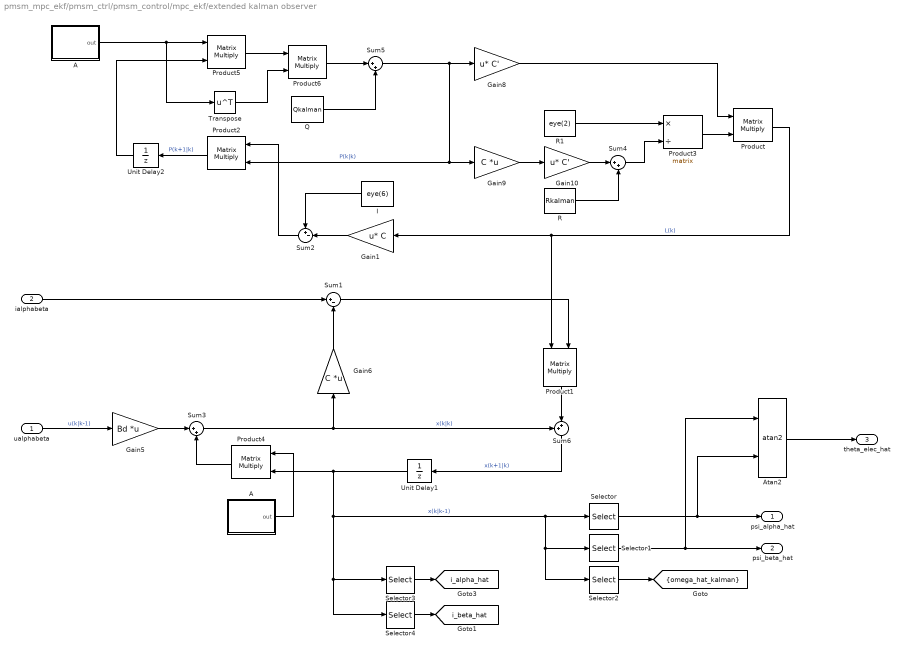
== system pmsm_mpc_ekf/pmsm_ctrl/pmsm_control/mpc_ekf/extended kalman observer ==
  ualphabeta : Inport
  ialphabeta : Inport  Port=2
  A : Subsystem
  "A " : Subsystem
  Atan2 : Trigonometry  Operator=atan2
  Gain1 : Gain  Gain=C  Multiplication=Matrix(u*K)
  Gain10 : Gain  Gain=C'  Multiplication=Matrix(u*K)
  Gain5 : Gain  Gain=Bd  Multiplication=Matrix(K*u)
  Gain6 : Gain  Gain=C  Multiplication=Matrix(K*u)
  Gain8 : Gain  Gain=C'  Multiplication=Matrix(u*K)
  Gain9 : Gain  Gain=C  Multiplication=Matrix(K*u)
  I : Constant  Value=eye(6)
  Product{,1..2,4..6} (6 alike) : Product  Multiplication=Matrix(*)
  Product3 : Product  Inputs=*/  Multiplication=Matrix(*)
  Q : Constant  Value=Qkalman
  R : Constant  Value=Rkalman
  R1 : Constant  Value=eye(2)
  Selector : Selector  InputPortWidth=6  IndexOptions=Index vector (dialog)  Indices=3  OutputSizes=1
  Selector1 : Selector  InputPortWidth=6  IndexOptions=Index vector (dialog)  Indices=4  OutputSizes=1
  Selector2 : Selector  InputPortWidth=6  IndexOptions=Index vector (dialog)  Indices=6  OutputSizes=1
  Selector3 : Selector  InputPortWidth=6  IndexOptions=Index vector (dialog)  Indices=1  OutputSizes=1
  Selector4 : Selector  InputPortWidth=6  IndexOptions=Index vector (dialog)  Indices=2  OutputSizes=1
  Sum1 : Sum  Inputs=|+-
  Sum2 : Sum  Inputs=+-|
  Sum3 : Sum  Inputs=|++
  Sum4 : Sum  Inputs=|++
  Sum5 : Sum  Inputs=|++
  Sum6 : Sum  Inputs=++|
  Transpose : Math  Operator=transpose
  Unit Delay1 : UnitDelay  InitialCondition=[0 0 tcontrol tcontrol 0 0]  SampleTime=tcontrol  HasFrameUpgradeWarning=on
  Unit Delay2 : UnitDelay  SampleTime=tcontrol  HasFrameUpgradeWarning=on
  psi_alpha_hat : Outport
  psi_beta_hat : Outport  Port=2
  theta_elec_hat : Outport  Port=3
  tag scope: i_alpha_hat=global, i_beta_hat=global, omega_hat_kalman=scoped
  wires:
  Gain5/1 -> Sum3/1
  Product4/1 -> Sum3/2
  Gain6/1 -> Sum1/2
  Sum5/1 -> Product2/2, Gain9/1, Gain8/1  "P(k|k)"
  Product5/1 -> Product6/1
  Product6/1 -> Sum5/1
  Q/1 -> Sum5/2
  Gain9/1 -> Gain10/1
  R/1 -> Sum4/2
  Gain10/1 -> Sum4/1
  Gain8/1 -> Product/1
  Product/1 -> Product1/1, Gain1/1  "L(k)"
  Product2/1 -> Unit Delay2/1  "P(k+1|k)"
  Sum2/1 -> Product2/1
  Unit Delay2/1 -> Product5/2
  Sum6/1 -> Unit Delay1/1  "x(k+1|k)"
  I/1 -> Sum2/1
  Gain1/1 -> Sum2/2
  Sum1/1 -> Product1/2
  ialphabeta/1 -> Sum1/1
  Sum4/1 -> Product3/2
  Product3/1 -> Product/2
  R1/1 -> Product3/1
  ualphabeta/1 -> Gain5/1  "u(k|k-1)"
  Sum3/1 -> Gain6/1, Sum6/1  "x(k|k)"
  Unit Delay1/1 -> Selector4/1, Selector3/1, Selector2/1, Selector1/1, Selector/1, Product4/2  "x(k|k-1)"
  A/1(out) -> Product4/1
  "A "/1(out) -> Transpose/1, Product5/1
  Product1/1 -> Sum6/2
  Selector1/1 -> Atan2/1, psi_beta_hat/1
  Selector/1 -> Atan2/2, psi_alpha_hat/1
  Transpose/1 -> Product6/2
  Selector2/1 -> [omega_hat_kalman]
  Selector3/1 -> [i_alpha_hat]
  Atan2/1 -> theta_elec_hat/1
  Selector4/1 -> [i_beta_hat]

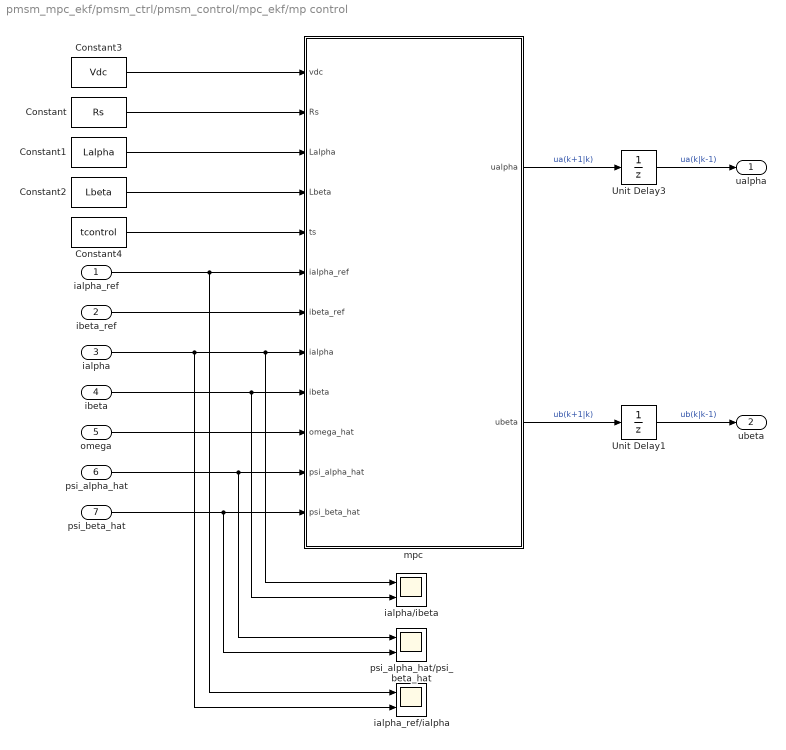
== system pmsm_mpc_ekf/pmsm_ctrl/pmsm_control/mpc_ekf/mp control ==
  ialpha_ref : Inport
  ibeta_ref : Inport  Port=2
  ialpha : Inport  Port=3
  ibeta : Inport  Port=4
  omega : Inport  Port=5
  psi_alpha_hat : Inport  Port=6
  psi_beta_hat : Inport  Port=7
  Constant : Constant  Value=Rs
  Constant1 : Constant  Value=Lalpha
  Constant2 : Constant  Value=Lbeta
  Constant3 : Constant  Value=Vdc
  Constant4 : Constant  Value=tcontrol
  Unit Delay1 : UnitDelay  SampleTime=tcontrol  HasFrameUpgradeWarning=on
  Unit Delay3 : UnitDelay  SampleTime=tcontrol  HasFrameUpgradeWarning=on
  ialpha/ibeta : Scope  NumInputPorts=2
      settings: SampleTime=ts  ActiveDisplayYMinimum=-1333.37712  ActiveDisplayYMaximum=1131.79846
  ialpha_ref/ialpha : Scope  NumInputPorts=2
      settings: SampleTime=ts  ActiveDisplayYMinimum=-1306.22726  ActiveDisplayYMaximum=1306.53939  DataLoggingVariableName=ScopeData2
  mpc : MATLAB Function  TreatAsAtomicUnit=on  SystemSampleTime=tcontrol
  psi_alpha_hat/psi_beta_hat : Scope  NumInputPorts=2
      settings: SampleTime=ts  ActiveDisplayYMinimum=-4.74729  ActiveDisplayYMaximum=4.18301
  ualpha : Outport
  ubeta : Outport  Port=2
  wires:
  Constant/1 -> mpc/2(Rs)
  ialpha_ref/1 -> mpc/6(ialpha_ref), ialpha_ref/ialpha/1
  ibeta_ref/1 -> mpc/7(ibeta_ref)
  Constant1/1 -> mpc/3(Lalpha)
  mpc/1(ualpha) -> Unit Delay3/1  "ua(k+1|k)"
  Unit Delay3/1 -> ualpha/1  "ua(k|k-1)"
  Constant3/1 -> mpc/1(vdc)
  Constant4/1 -> mpc/5(ts)
  ialpha/1 -> ialpha/ibeta/1, mpc/8(ialpha), ialpha_ref/ialpha/2
  ibeta/1 -> ialpha/ibeta/2, mpc/9(ibeta)
  Unit Delay1/1 -> ubeta/1  "ub(k|k-1)"
  mpc/2(ubeta) -> Unit Delay1/1  "ub(k+1|k)"
  omega/1 -> mpc/10(omega_hat)
  psi_alpha_hat/1 -> psi_alpha_hat/psi_beta_hat/1, mpc/11(psi_alpha_hat)
  psi_beta_hat/1 -> mpc/12(psi_beta_hat), psi_alpha_hat/psi_beta_hat/2
  Constant2/1 -> mpc/4(Lbeta)

== system pmsm_mpc_ekf/psm_mpc/pmsm_control/mpc_ekf/current_reference_generator ==
  torque_ref_pu : Inport
  theta_elec_hat : Inport  Port=2
  Gain5 : Gain  Gain=-1
  Gain6 : Gain  Gain=ibez
  Product : Product
  Product1 : Product
  Trigonometric Function1 : Trigonometry
  Trigonometric Function2 : Trigonometry  Operator=cos
  i_alpha_ref : Outport
  i_beta_ref : Outport  Port=2
  wires:
  torque_ref_pu/1 -> Gain6/1
  Trigonometric Function1/1 -> Product/2
  Product1/1 -> i_beta_ref/1
  Trigonometric Function2/1 -> Product1/2
  Product/1 -> Gain5/1
  Gain5/1 -> i_alpha_ref/1
  Gain6/1 -> Product/1, Product1/1
  theta_elec_hat/1 -> Trigonometric Function1/1, Trigonometric Function2/1  "theta_electrical"

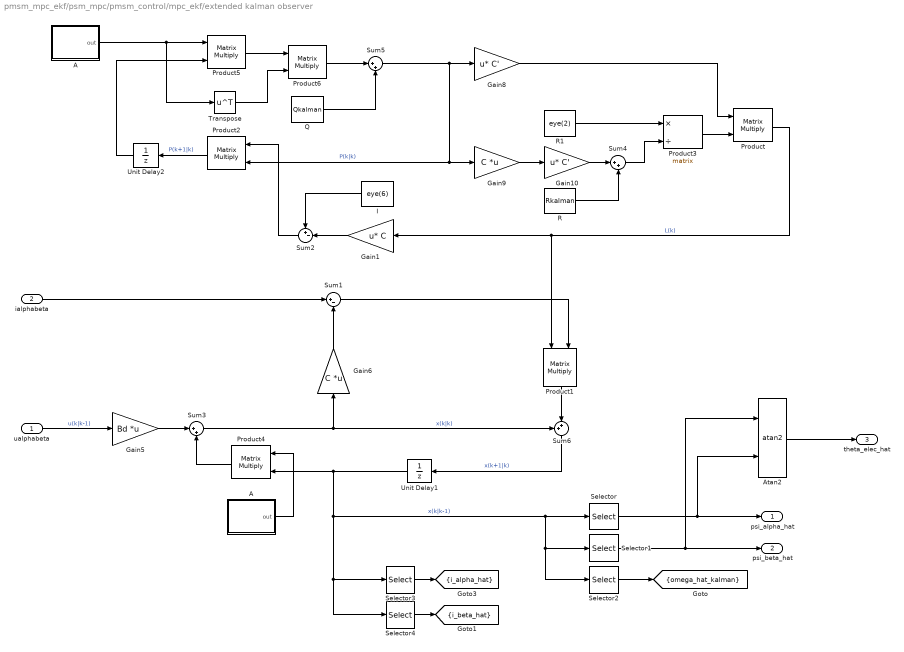
== system pmsm_mpc_ekf/psm_mpc/pmsm_control/mpc_ekf/extended kalman observer ==
  ualphabeta : Inport
  ialphabeta : Inport  Port=2
  A : Subsystem
  "A " : Subsystem
  Atan2 : Trigonometry  Operator=atan2
  Gain1 : Gain  Gain=C  Multiplication=Matrix(u*K)
  Gain10 : Gain  Gain=C'  Multiplication=Matrix(u*K)
  Gain5 : Gain  Gain=Bd  Multiplication=Matrix(K*u)
  Gain6 : Gain  Gain=C  Multiplication=Matrix(K*u)
  Gain8 : Gain  Gain=C'  Multiplication=Matrix(u*K)
  Gain9 : Gain  Gain=C  Multiplication=Matrix(K*u)
  I : Constant  Value=eye(6)
  Product{,1..2,4..6} (6 alike) : Product  Multiplication=Matrix(*)
  Product3 : Product  Inputs=*/  Multiplication=Matrix(*)
  Q : Constant  Value=Qkalman
  R : Constant  Value=Rkalman
  R1 : Constant  Value=eye(2)
  Selector : Selector  InputPortWidth=6  IndexOptions=Index vector (dialog)  Indices=3  OutputSizes=1
  Selector1 : Selector  InputPortWidth=6  IndexOptions=Index vector (dialog)  Indices=4  OutputSizes=1
  Selector2 : Selector  InputPortWidth=6  IndexOptions=Index vector (dialog)  Indices=6  OutputSizes=1
  Selector3 : Selector  InputPortWidth=6  IndexOptions=Index vector (dialog)  Indices=1  OutputSizes=1
  Selector4 : Selector  InputPortWidth=6  IndexOptions=Index vector (dialog)  Indices=2  OutputSizes=1
  Sum1 : Sum  Inputs=|+-
  Sum2 : Sum  Inputs=+-|
  Sum3 : Sum  Inputs=|++
  Sum4 : Sum  Inputs=|++
  Sum5 : Sum  Inputs=|++
  Sum6 : Sum  Inputs=++|
  Transpose : Math  Operator=transpose
  Unit Delay1 : UnitDelay  InitialCondition=[0 0 tcontrol tcontrol 0 0]  SampleTime=tcontrol  HasFrameUpgradeWarning=on
  Unit Delay2 : UnitDelay  SampleTime=tcontrol  HasFrameUpgradeWarning=on
  psi_alpha_hat : Outport
  psi_beta_hat : Outport  Port=2
  theta_elec_hat : Outport  Port=3
  tag scope: i_alpha_hat=scoped, i_beta_hat=scoped, omega_hat_kalman=scoped
  wires:
  Selector4/1 -> [i_beta_hat]
  Atan2/1 -> theta_elec_hat/1
  Selector3/1 -> [i_alpha_hat]
  Selector2/1 -> [omega_hat_kalman]
  Transpose/1 -> Product6/2
  Selector/1 -> psi_alpha_hat/1, Atan2/2
  Selector1/1 -> psi_beta_hat/1, Atan2/1
  Product1/1 -> Sum6/2
  "A "/1(out) -> Product5/1, Transpose/1
  A/1(out) -> Product4/1
  Unit Delay1/1 -> Product4/2, Selector/1, Selector1/1, Selector2/1, Selector3/1, Selector4/1  "x(k|k-1)"
  Sum3/1 -> Sum6/1, Gain6/1  "x(k|k)"
  ualphabeta/1 -> Gain5/1  "u(k|k-1)"
  R1/1 -> Product3/1
  Product3/1 -> Product/2
  Sum4/1 -> Product3/2
  ialphabeta/1 -> Sum1/1
  Sum1/1 -> Product1/2
  Gain1/1 -> Sum2/2
  I/1 -> Sum2/1
  Sum6/1 -> Unit Delay1/1  "x(k+1|k)"
  Unit Delay2/1 -> Product5/2
  Sum2/1 -> Product2/1
  Product2/1 -> Unit Delay2/1  "P(k+1|k)"
  Product/1 -> Gain1/1, Product1/1  "L(k)"
  Gain8/1 -> Product/1
  Gain10/1 -> Sum4/1
  R/1 -> Sum4/2
  Gain9/1 -> Gain10/1
  Q/1 -> Sum5/2
  Product6/1 -> Sum5/1
  Product5/1 -> Product6/1
  Sum5/1 -> Gain8/1, Gain9/1, Product2/2  "P(k|k)"
  Gain6/1 -> Sum1/2
  Product4/1 -> Sum3/2
  Gain5/1 -> Sum3/1
